simulink library "mspread"  (Simulink 6.0)
settings: Solver=ode45  SolverMode=SingleTasking  StartTime=0.0  StopTime=10.0  RelTol=1e-3
libraries: dspsigops x4, commfilt2 x3, commdigbbndpm2 x2, dspmtrx3 x1, dspsigattribs x1, dspsrcs4 x1
settings Model: Creator=akansal  LastModifiedBy=akansal  ExtModeAutoUpdateStatusClock=off  ProdHWDeviceType=Specified
settings DataIOCC: SignalLoggingName=logsOut
settings OptimizationCC: BooleanDataType=off
settings DebuggingCC: CheckExecutionContextPreStartOutputMsg=on  CheckExecutionContextRuntimeOutputMsg=on  SolverPrmCheckMsg=none
settings HardwareCC: ProdHWDeviceType=Specified
settings ModelReferenceCC: UpdateModelReferenceTargets=IfOutOfDate
settings GRTTargetCC: LifeSpan=inf
settings SFSimCC: SFSimApplyToAllLibs=on  SFSimBuildMode=Incremental

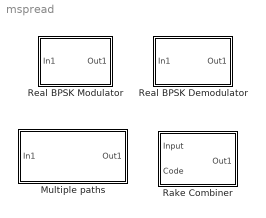
== system mspread ==
  Multiple paths : Subsystem  EnableExecutionContextPropagation=on  mask(Multiple Paths){p=3, pd=[0 2 6], ts=1/19200}
      mask prompts: p "Number of paths:"; pd "Path delays:"; ts "Input sample time:"
      mask help: The input signal traverses through the multiple paths and the output is a combined signal.
      mask Display: disp(['Propagate through \n' num2str(p) ' Paths']);
  Rake Combiner : Subsystem  EnableExecutionContextPropagation=on  mask(Rake combiner){pd=[0 2 6], pgain=64}
      mask prompts: pd "Delay vector (in samples for 3 paths):"; pgain "Samples to integrate:"
      mask help: The individual paths are equally combined in terms of power/gain.
      mask Display: disp('Rake\nCombiner');
  Real BPSK Demodulator : Subsystem  EnableExecutionContextPropagation=on
      mask Type: Real BPSK Demodulator
      mask Display: disp('Real BPSK\nDemodulator');
  Real BPSK Modulator : Subsystem  EnableExecutionContextPropagation=on
      mask Type: Real BPSK Modulator
      mask Display: disp('Real BPSK\nModulator');

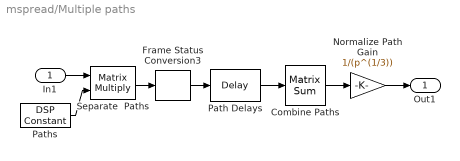
== system mspread/Multiple paths ==
  In1 : Inport  LatchInput=off
  Combine Paths : dspmtrx3/Matrix Sum  Dim=Rows  roundingMode=Floor  overflowMode=off
  Frame Status Conversion3 : dspsigattribs/Frame Status Conversion  growRefPort=off  outframe=Frame-based
  Normalize Path Gain : Gain  Gain=1/(p^(1/3))  SaturateOnIntegerOverflow=on
  Path Delays : dspsigops/Delay  dly_unit=Samples  delay=pd  ic_detail=off  dif_ic_for_ch=off  dif_ic_for_dly=off  ic=0  reset_popup=None
  Paths : dspsrcs4/DSP Constant  Value=ones(1,p)  SampleMode=Discrete  discreteOutput=Frame-based  continuousOutput=Sample-based  sampTime=ts  framePeriod=ts  dataType=Inherit from 'Constant value'  wordLen=16  udDataType=sfix(16)  fracBitsMode=Best precision  numFracBits=15  InterpretAs1D=off  Ts=ts  FramebasedOutput=on
  Separate  Paths : Product  Multiplication=Matrix(*)  SaturateOnIntegerOverflow=on  InputSameDT=on
  Out1 : Outport
  wires:
  Normalize Path Gain/1 -> Out1/1
  In1/1 -> Separate  Paths/1
  Combine Paths/1 -> Normalize Path Gain/1
  Path Delays/1 -> Combine Paths/1
  Separate  Paths/1 -> Frame Status Conversion3/1
  Paths/1 -> Separate  Paths/2
  Frame Status Conversion3/1 -> Path Delays/1

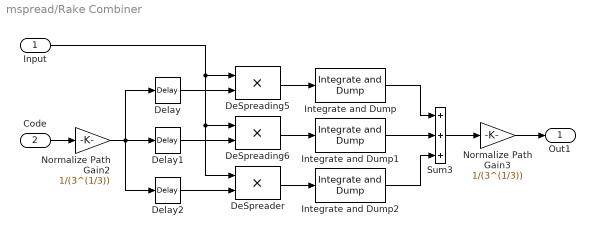
== system mspread/Rake Combiner ==
  Input : Inport  LatchInput=off
  Code : Inport  Port=2  LatchInput=off
  DeSpreader : Product  SaturateOnIntegerOverflow=on  InputSameDT=on
  DeSpreading5 : Product  SaturateOnIntegerOverflow=on  InputSameDT=on
  DeSpreading6 : Product  SaturateOnIntegerOverflow=on  InputSameDT=on
  Delay : dspsigops/Delay  dly_unit=Samples  delay=pd(1)  ic_detail=off  dif_ic_for_ch=off  dif_ic_for_dly=off  ic=0  reset_popup=None
  Delay1 : dspsigops/Delay  dly_unit=Samples  delay=pd(2)  ic_detail=off  dif_ic_for_ch=off  dif_ic_for_dly=off  ic=0  reset_popup=None
  Delay2 : dspsigops/Delay  dly_unit=Samples  delay=pd(3)  ic_detail=off  dif_ic_for_ch=off  dif_ic_for_dly=off  ic=0  reset_popup=None
  Integrate and Dump : commfilt2/Integrate and Dump  obssamples=pgain  offsetsamples=0  nodump=off
  Integrate and Dump1 : commfilt2/Integrate and Dump  obssamples=pgain  offsetsamples=0  nodump=off
  Integrate and Dump2 : commfilt2/Integrate and Dump  obssamples=pgain  offsetsamples=0  nodump=off
  Normalize Path Gain2 : Gain  Gain=1/(3^(1/3))  SaturateOnIntegerOverflow=on
  Normalize Path Gain3 : Gain  Gain=1/(3^(1/3))  SaturateOnIntegerOverflow=on
  Sum3 : Sum  Inputs=+++  SaturateOnIntegerOverflow=on  InputSameDT=on
  Out1 : Outport
  wires:
  DeSpreading5/1 -> Integrate and Dump/1
  DeSpreading6/1 -> Integrate and Dump1/1
  DeSpreader/1 -> Integrate and Dump2/1
  Integrate and Dump1/1 -> Sum3/2
  Integrate and Dump2/1 -> Sum3/3
  Integrate and Dump/1 -> Sum3/1
  Sum3/1 -> Normalize Path Gain3/1
  Normalize Path Gain3/1 -> Out1/1
  Delay/1 -> DeSpreading5/2
  Delay1/1 -> DeSpreading6/2
  Delay2/1 -> DeSpreader/2
  Normalize Path Gain2/1 -> Delay/1, Delay1/1, Delay2/1
  Code/1 -> Normalize Path Gain2/1
  Input/1 -> DeSpreader/1, DeSpreading6/1, DeSpreading5/1

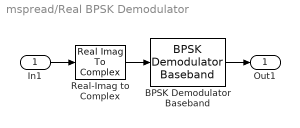
== system mspread/Real BPSK Demodulator ==
  In1 : Inport  LatchInput=off
  BPSK Demodulator Baseband : commdigbbndpm2/BPSK Demodulator Baseband  Ph=0  numSamp=1
  Real-Imag to Complex : RealImagToComplex  Input=Real
  Out1 : Outport
  wires:
  Real-Imag to Complex/1 -> BPSK Demodulator Baseband/1
  BPSK Demodulator Baseband/1 -> Out1/1
  In1/1 -> Real-Imag to Complex/1

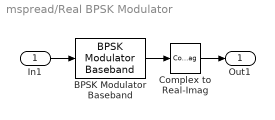
== system mspread/Real BPSK Modulator ==
  In1 : Inport  LatchInput=off
  BPSK Modulator Baseband : commdigbbndpm2/BPSK Modulator Baseband  Ph=0  numSamp=1
  Complex to Real-Imag : ComplexToRealImag  Output=Real
  Out1 : Outport
  wires:
  BPSK Modulator Baseband/1 -> Complex to Real-Imag/1
  In1/1 -> BPSK Modulator Baseband/1
  Complex to Real-Imag/1 -> Out1/1
